simulink model "powerwindow_tl"  (R2018b)
settings: Solver=ode3  StartTime=0.0  StopTime=inf  FixedStep=0.01  RelTol=1e-3  EnableMultiTasking=on
PreLoadFcn:
  | if exist('tl_preloadfcn','file'), tl_preloadfcn(gcs,'4.4.0.41'); end
PostLoadFcn:
  | , if any(exist('dsrtsu_mdlpostloadfcn', 'file') == [2, 3, 6]), try dsrtsu_mdlpostloadfcn('Execute', bdroot); catch fprintf('Error in PostLoadFcn (dsrtsu_mdlpostloadfcn) for model "%s":\n %s\n', bdroot, lasterr); end, end,
  | if exist('tl_postloadfcn','file'), tl_postloadfcn(gcs,'4.4.0.41'); end
InitFcn:
  | if exist('tlds_init','file'), tlds_init(gcs); end
StartFcn:
  | if exist('tlds_start','file'), tlds_start(gcs); end
StopFcn:
  | if exist('tlds_stop','file'), tlds_stop(gcs); end
model workspace (MAT data in the model file):
  obs_1 = 1
  obs_10 = 1
  obs_11 = 1
  obs_12 = 1
  obs_13 = 1
  obs_14 = 1
  obs_15 = 1
  obs_16 = 1
  obs_17 = 1
  obs_18 = 1
  obs_19 = 1
  obs_2 = 1
  obs_20 = 1
  obs_21 = 1
  obs_22 = 1
  obs_23 = 1
  obs_24 = 1
  obs_25 = 1
  obs_26 = 1
  obs_27 = 1
  obs_28 = 1
  obs_29 = 1
  obs_3 = 1
  obs_30 = 1
  obs_31 = 1
  obs_32 = 1
  obs_4 = 1
  obs_5 = 1
  obs_6 = 1
  obs_7 = 1
  obs_8 = 1
  obs_9 = 1
values from neighbouring files (symbols this model uses):
  auto_down_time = 100    [start.m]
  auto_up_time = 100    [start.m]
  emergency_down_time = 100    [start.m]
  position_endstop_top = 0.4    [start.m]
undefined symbols (not defined in the file or in its folder): DiscIntNeverNeededParam
libraries: tllib x5
(part 2 of 2)

== system powerwindow_tl/PowerWindowController/Subsystem/PowerWindowController/detect_obstacle_endstop/detect_endstop ==
  window_position : Inport
  detection_ endstop_bottom : RelationalOperator  Operator=<=  OutDataTypeStr=boolean  RndMeth=Nearest  InputSameDT=on  mask(TL_RelationalOperator){data={'date',736551.40566996532}}
      settings: CopyFcn=if exist('copy_tlblock','file')==2,copy_tlblock(gcbh);end  DeleteFcn=if exist('delete_tlblock','file')==2,delete_tlblock(gcbh);end  NameChangeFcn=if exist('rename_tlblock','file')==2,rename_tlblock(gcbh);end  OpenFcn=if exist('tl_open_blockdlg','file')==2,tl_open_blockdlg(gcbh);else,open_system(gcbh,'parameter');end
      mask Help: eval(['if exist(''tl_online_help'',''file'') == 2, tl_online_help(''Topic'',''TL_RelationalOperator''),else, web([''jar:file:///'',matlabroot,''/help/toolbox/simulink/help.jar!/slref/' lower(get_param(gcbh,'Blocktype')) '.html''], ''-helpbrowser''),end'])
      mask Display:
      | [x,y] = tlDrawBrandOnBlockIcon(gcbh);
      | plot(x,y);
  detection_ endstop_top : RelationalOperator  OutDataTypeStr=boolean  RndMeth=Nearest  InputSameDT=on  mask(TL_RelationalOperator){data={'date',736551.40567012737}}
      settings: CopyFcn=if exist('copy_tlblock','file')==2,copy_tlblock(gcbh);end  DeleteFcn=if exist('delete_tlblock','file')==2,delete_tlblock(gcbh);end  NameChangeFcn=if exist('rename_tlblock','file')==2,rename_tlblock(gcbh);end  OpenFcn=if exist('tl_open_blockdlg','file')==2,tl_open_blockdlg(gcbh);else,open_system(gcbh,'parameter');end
      mask Help: eval(['if exist(''tl_online_help'',''file'') == 2, tl_online_help(''Topic'',''TL_RelationalOperator''),else, web([''jar:file:///'',matlabroot,''/help/toolbox/simulink/help.jar!/slref/' lower(get_param(gcbh,'Blocktype')) '.html''], ''-helpbrowser''),end'])
      mask Display:
      | [x,y] = tlDrawBrandOnBlockIcon(gcbh);
      | plot(x,y);
  position_ endstop_bottom : Constant  Value=0  mask(TL_Constant){data={'date',736551.40567030094}}
      settings: CopyFcn=if exist('copy_tlblock','file')==2,copy_tlblock(gcbh);end  DeleteFcn=if exist('delete_tlblock','file')==2,delete_tlblock(gcbh);end  NameChangeFcn=if exist('rename_tlblock','file')==2,rename_tlblock(gcbh);end  OpenFcn=if exist('tl_open_blockdlg','file')==2,tl_open_blockdlg(gcbh);else,open_system(gcbh,'parameter');end
      mask Help: eval(['if exist(''tl_online_help'',''file'') == 2, tl_online_help(''Topic'',''TL_Constant''),else, web([''jar:file:///'',matlabroot,''/help/toolbox/simulink/help.jar!/slref/' lower(get_param(gcbh,'Blocktype')) '.html''], ''-helpbrowser''),end'])
      mask Display:
      | [x,y] = tlDrawBrandOnBlockIcon(gcbh);
      | plot(x,y);
  position_ endstop_top : Constant  Value=position_endstop_top  mask(TL_Constant){data={'output',{'variable','position_endstop_top'},'date',736551.4102625231}}
      settings: CopyFcn=if exist('copy_tlblock','file')==2,copy_tlblock(gcbh);end  DeleteFcn=if exist('delete_tlblock','file')==2,delete_tlblock(gcbh);end  NameChangeFcn=if exist('rename_tlblock','file')==2,rename_tlblock(gcbh);end  OpenFcn=if exist('tl_open_blockdlg','file')==2,tl_open_blockdlg(gcbh);else,open_system(gcbh,'parameter');end
      mask Help: eval(['if exist(''tl_online_help'',''file'') == 2, tl_online_help(''Topic'',''TL_Constant''),else, web([''jar:file:///'',matlabroot,''/help/toolbox/simulink/help.jar!/slref/' lower(get_param(gcbh,'Blocktype')) '.html''], ''-helpbrowser''),end'])
      mask Display:
      | [x,y] = tlDrawBrandOnBlockIcon(gcbh);
      | plot(x,y);
  endstop_top : Outport
  endstop_bottom : Outport  Port=2
  wires:
  position_ endstop_top/1 -> detection_ endstop_top/2
  detection_ endstop_bottom/1 -> endstop_bottom/1  "endstop_bottom"
  detection_ endstop_top/1 -> endstop_top/1  "endstop_top"
  window_position/1 -> detection_ endstop_top/1, detection_ endstop_bottom/1
  position_ endstop_bottom/1 -> detection_ endstop_bottom/2

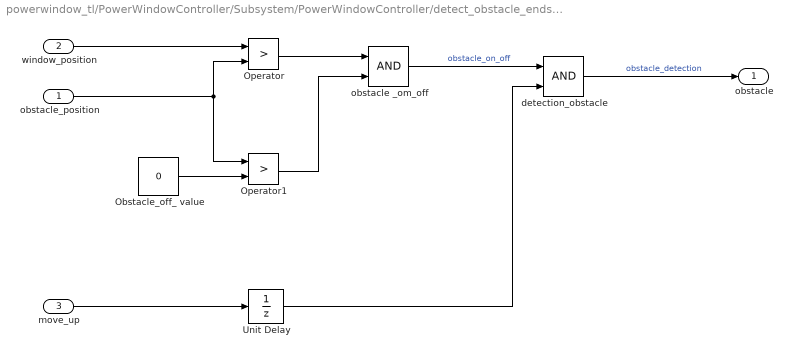
== system powerwindow_tl/PowerWindowController/Subsystem/PowerWindowController/detect_obstacle_endstop/detect_obstacle ==
  obstacle_position : Inport
  window_position : Inport  Port=2
  move_up : Inport  Port=3
  Obstacle_off_ value : Constant  Value=0  mask(TL_Constant){data={'date',736551.40567067126}}
      settings: CopyFcn=if exist('copy_tlblock','file')==2,copy_tlblock(gcbh);end  DeleteFcn=if exist('delete_tlblock','file')==2,delete_tlblock(gcbh);end  NameChangeFcn=if exist('rename_tlblock','file')==2,rename_tlblock(gcbh);end  OpenFcn=if exist('tl_open_blockdlg','file')==2,tl_open_blockdlg(gcbh);else,open_system(gcbh,'parameter');end
      mask Help: eval(['if exist(''tl_online_help'',''file'') == 2, tl_online_help(''Topic'',''TL_Constant''),else, web([''jar:file:///'',matlabroot,''/help/toolbox/simulink/help.jar!/slref/' lower(get_param(gcbh,'Blocktype')) '.html''], ''-helpbrowser''),end'])
      mask Display:
      | [x,y] = tlDrawBrandOnBlockIcon(gcbh);
      | plot(x,y);
  Operator : RelationalOperator  Operator=>  OutDataTypeStr=boolean  RndMeth=Nearest  InputSameDT=on  mask(TL_RelationalOperator){data={'date',736551.40567081014}}
      settings: CopyFcn=if exist('copy_tlblock','file')==2,copy_tlblock(gcbh);end  DeleteFcn=if exist('delete_tlblock','file')==2,delete_tlblock(gcbh);end  NameChangeFcn=if exist('rename_tlblock','file')==2,rename_tlblock(gcbh);end  OpenFcn=if exist('tl_open_blockdlg','file')==2,tl_open_blockdlg(gcbh);else,open_system(gcbh,'parameter');end
      mask Help: eval(['if exist(''tl_online_help'',''file'') == 2, tl_online_help(''Topic'',''TL_RelationalOperator''),else, web([''jar:file:///'',matlabroot,''/help/toolbox/simulink/help.jar!/slref/' lower(get_param(gcbh,'Blocktype')) '.html''], ''-helpbrowser''),end'])
      mask Display:
      | [x,y] = tlDrawBrandOnBlockIcon(gcbh);
      | plot(x,y);
  Operator1 : RelationalOperator  Operator=>  OutDataTypeStr=boolean  RndMeth=Nearest  InputSameDT=on  mask(TL_RelationalOperator){data={'date',736551.40567097219}}
      settings: CopyFcn=if exist('copy_tlblock','file')==2,copy_tlblock(gcbh);end  DeleteFcn=if exist('delete_tlblock','file')==2,delete_tlblock(gcbh);end  NameChangeFcn=if exist('rename_tlblock','file')==2,rename_tlblock(gcbh);end  OpenFcn=if exist('tl_open_blockdlg','file')==2,tl_open_blockdlg(gcbh);else,open_system(gcbh,'parameter');end
      mask Help: eval(['if exist(''tl_online_help'',''file'') == 2, tl_online_help(''Topic'',''TL_RelationalOperator''),else, web([''jar:file:///'',matlabroot,''/help/toolbox/simulink/help.jar!/slref/' lower(get_param(gcbh,'Blocktype')) '.html''], ''-helpbrowser''),end'])
      mask Display:
      | [x,y] = tlDrawBrandOnBlockIcon(gcbh);
      | plot(x,y);
  Unit Delay : UnitDelay  SampleTime=-1  mask(TL_UnitDelay){data={'output',{'variable','move_up_cmd'},'state',{'type','Bool'},'date',737383.60909223382}}
      settings: CopyFcn=if exist('copy_tlblock','file')==2,copy_tlblock(gcbh);end  DeleteFcn=if exist('delete_tlblock','file')==2,delete_tlblock(gcbh);end  NameChangeFcn=if exist('rename_tlblock','file')==2,rename_tlblock(gcbh);end  OpenFcn=if exist('tl_open_blockdlg','file')==2,tl_open_blockdlg(gcbh);else,open_system(gcbh,'parameter');end
      mask Help: eval(['if exist(''tl_online_help'',''file'') == 2, tl_online_help(''Topic'',''TL_UnitDelay''),else, web([''jar:file:///'',matlabroot,''/help/toolbox/simulink/help.jar!/slref/' lower(get_param(gcbh,'Blocktype')) '.html''], ''-helpbrowser''),end'])
      mask Display:
      | [x,y] = tlDrawBrandOnBlockIcon(gcbh);
      | plot(x,y);
  detection_obstacle : Logic  AllPortsSameDT=off  OutDataTypeStr=boolean  mask(TL_LogicalOperator){data={'date',736551.40567170142}}
      settings: CopyFcn=if exist('copy_tlblock','file')==2,copy_tlblock(gcbh);end  DeleteFcn=if exist('delete_tlblock','file')==2,delete_tlblock(gcbh);end  NameChangeFcn=if exist('rename_tlblock','file')==2,rename_tlblock(gcbh);end  OpenFcn=if exist('tl_open_blockdlg','file')==2,tl_open_blockdlg(gcbh);else,open_system(gcbh,'parameter');end
      mask Help: eval(['if exist(''tl_online_help'',''file'') == 2, tl_online_help(''Topic'',''TL_LogicalOperator''),else, web([''jar:file:///'',matlabroot,''/help/toolbox/simulink/help.jar!/slref/' lower(get_param(gcbh,'Blocktype')) '.html''], ''-helpbrowser''),end'])
      mask Display:
      | [x,y] = tlDrawBrandOnBlockIcon(gcbh);
      | plot(x,y);
  obstacle _om_off : Logic  AllPortsSameDT=off  OutDataTypeStr=boolean  mask(TL_LogicalOperator){data={'date',736551.40567187499}}
      settings: CopyFcn=if exist('copy_tlblock','file')==2,copy_tlblock(gcbh);end  DeleteFcn=if exist('delete_tlblock','file')==2,delete_tlblock(gcbh);end  NameChangeFcn=if exist('rename_tlblock','file')==2,rename_tlblock(gcbh);end  OpenFcn=if exist('tl_open_blockdlg','file')==2,tl_open_blockdlg(gcbh);else,open_system(gcbh,'parameter');end
      mask Help: eval(['if exist(''tl_online_help'',''file'') == 2, tl_online_help(''Topic'',''TL_LogicalOperator''),else, web([''jar:file:///'',matlabroot,''/help/toolbox/simulink/help.jar!/slref/' lower(get_param(gcbh,'Blocktype')) '.html''], ''-helpbrowser''),end'])
      mask Display:
      | [x,y] = tlDrawBrandOnBlockIcon(gcbh);
      | plot(x,y);
  obstacle : Outport
  wires:
  obstacle _om_off/1 -> detection_obstacle/1  "obstacle_on_off"
  Obstacle_off_ value/1 -> Operator1/2
  Operator1/1 -> obstacle _om_off/2
  detection_obstacle/1 -> obstacle/1  "obstacle_detection"
  Unit Delay/1 -> detection_obstacle/2
  obstacle_position/1 -> Operator1/1, Operator/2
  move_up/1 -> Unit Delay/1
  window_position/1 -> Operator/1
  Operator/1 -> obstacle _om_off/1

== system powerwindow_tl/PowerWindowController/Subsystem/PowerWindowController/validate_driver/check_down ==
  action : Inport
  endstop : Inport  Port=2
  allow_action : Logic  mask(TL_LogicalOperator){data={'date',736551.40567218745}}
      settings: DeleteFcn=if exist('delete_tlblock','file')==2,delete_tlblock(gcbh);end  NameChangeFcn=if exist('rename_tlblock','file')==2,rename_tlblock(gcbh);end  OpenFcn=if exist('tl_open_blockdlg','file')==2,tl_open_blockdlg(gcbh);else,open_system(gcbh,'parameter');end
      mask Help: eval(['if exist(''tl_online_help'',''file'') == 2, tl_online_help(''Topic'',''TL_LogicalOperator''),else, web([''jar:file:///'',matlabroot,''/help/toolbox/simulink/help.jar!/slref/' lower(get_param(gcbh,'Blocktype')) '.html''], ''-helpbrowser''),end'])
      mask Display: plot([-0.05, 1.05, NaN, -0.05, 1.05],[.01, .01, NaN, .99, .99])
  not : Logic  Operator=NOT  Inputs=1  mask(TL_LogicalOperator){data={'date',736551.40567231481}}
      settings: DeleteFcn=if exist('delete_tlblock','file')==2,delete_tlblock(gcbh);end  NameChangeFcn=if exist('rename_tlblock','file')==2,rename_tlblock(gcbh);end  OpenFcn=if exist('tl_open_blockdlg','file')==2,tl_open_blockdlg(gcbh);else,open_system(gcbh,'parameter');end
      mask Help: eval(['if exist(''tl_online_help'',''file'') == 2, tl_online_help(''Topic'',''TL_LogicalOperator''),else, web([''jar:file:///'',matlabroot,''/help/toolbox/simulink/help.jar!/slref/' lower(get_param(gcbh,'Blocktype')) '.html''], ''-helpbrowser''),end'])
      mask Display: plot([-0.05, 1.05, NaN, -0.05, 1.05],[.01, .01, NaN, .99, .99])
  checked_action : Outport
  wires:
  not/1 -> allow_action/2
  action/1 -> allow_action/1
  allow_action/1 -> checked_action/1  "checked_action"
  endstop/1 -> not/1

== system powerwindow_tl/PowerWindowController/Subsystem/PowerWindowController/validate_driver/check_up ==
  action : Inport
  endstop : Inport  Port=2
  allow_action : Logic  mask(TL_LogicalOperator){data={'date',736551.40567245369}}
      settings: DeleteFcn=if exist('delete_tlblock','file')==2,delete_tlblock(gcbh);end  NameChangeFcn=if exist('rename_tlblock','file')==2,rename_tlblock(gcbh);end  OpenFcn=if exist('tl_open_blockdlg','file')==2,tl_open_blockdlg(gcbh);else,open_system(gcbh,'parameter');end
      mask Help: eval(['if exist(''tl_online_help'',''file'') == 2, tl_online_help(''Topic'',''TL_LogicalOperator''),else, web([''jar:file:///'',matlabroot,''/help/toolbox/simulink/help.jar!/slref/' lower(get_param(gcbh,'Blocktype')) '.html''], ''-helpbrowser''),end'])
      mask Display: plot([-0.05, 1.05, NaN, -0.05, 1.05],[.01, .01, NaN, .99, .99])
  not : Logic  Operator=NOT  Inputs=1  mask(TL_LogicalOperator){data={'date',736551.40567262727}}
      settings: DeleteFcn=if exist('delete_tlblock','file')==2,delete_tlblock(gcbh);end  NameChangeFcn=if exist('rename_tlblock','file')==2,rename_tlblock(gcbh);end  OpenFcn=if exist('tl_open_blockdlg','file')==2,tl_open_blockdlg(gcbh);else,open_system(gcbh,'parameter');end
      mask Help: eval(['if exist(''tl_online_help'',''file'') == 2, tl_online_help(''Topic'',''TL_LogicalOperator''),else, web([''jar:file:///'',matlabroot,''/help/toolbox/simulink/help.jar!/slref/' lower(get_param(gcbh,'Blocktype')) '.html''], ''-helpbrowser''),end'])
      mask Display: plot([-0.05, 1.05, NaN, -0.05, 1.05],[.01, .01, NaN, .99, .99])
  checked_action : Outport
  wires:
  endstop/1 -> not/1
  allow_action/1 -> checked_action/1  "checked_action"
  action/1 -> allow_action/1
  not/1 -> allow_action/2

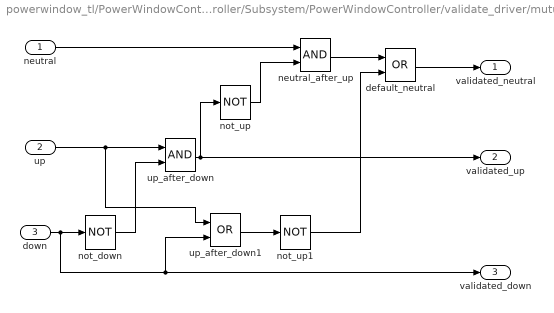
== system powerwindow_tl/PowerWindowController/Subsystem/PowerWindowController/validate_driver/mutually_exclusive ==
  neutral : Inport
  up : Inport  Port=2
  down : Inport  Port=3
  default_neutral : Logic  Operator=OR  mask(TL_LogicalOperator){data={'date',736551.40567276615}}
      settings: DeleteFcn=if exist('delete_tlblock','file')==2,delete_tlblock(gcbh);end  NameChangeFcn=if exist('rename_tlblock','file')==2,rename_tlblock(gcbh);end  OpenFcn=if exist('tl_open_blockdlg','file')==2,tl_open_blockdlg(gcbh);else,open_system(gcbh,'parameter');end
      mask Help: eval(['if exist(''tl_online_help'',''file'') == 2, tl_online_help(''Topic'',''TL_LogicalOperator''),else, web([''jar:file:///'',matlabroot,''/help/toolbox/simulink/help.jar!/slref/' lower(get_param(gcbh,'Blocktype')) '.html''], ''-helpbrowser''),end'])
      mask Display: plot([-0.05, 1.05, NaN, -0.05, 1.05],[.01, .01, NaN, .99, .99])
  neutral_after_up : Logic  mask(TL_LogicalOperator){data={'date',736551.40567293984}}
      settings: DeleteFcn=if exist('delete_tlblock','file')==2,delete_tlblock(gcbh);end  NameChangeFcn=if exist('rename_tlblock','file')==2,rename_tlblock(gcbh);end  OpenFcn=if exist('tl_open_blockdlg','file')==2,tl_open_blockdlg(gcbh);else,open_system(gcbh,'parameter');end
      mask Help: eval(['if exist(''tl_online_help'',''file'') == 2, tl_online_help(''Topic'',''TL_LogicalOperator''),else, web([''jar:file:///'',matlabroot,''/help/toolbox/simulink/help.jar!/slref/' lower(get_param(gcbh,'Blocktype')) '.html''], ''-helpbrowser''),end'])
      mask Display: plot([-0.05, 1.05, NaN, -0.05, 1.05],[.01, .01, NaN, .99, .99])
  not_down : Logic  Operator=NOT  Inputs=1  mask(TL_LogicalOperator){data={'date',736551.40567306709}}
      settings: DeleteFcn=if exist('delete_tlblock','file')==2,delete_tlblock(gcbh);end  NameChangeFcn=if exist('rename_tlblock','file')==2,rename_tlblock(gcbh);end  OpenFcn=if exist('tl_open_blockdlg','file')==2,tl_open_blockdlg(gcbh);else,open_system(gcbh,'parameter');end
      mask Help: eval(['if exist(''tl_online_help'',''file'') == 2, tl_online_help(''Topic'',''TL_LogicalOperator''),else, web([''jar:file:///'',matlabroot,''/help/toolbox/simulink/help.jar!/slref/' lower(get_param(gcbh,'Blocktype')) '.html''], ''-helpbrowser''),end'])
      mask Display: plot([-0.05, 1.05, NaN, -0.05, 1.05],[.01, .01, NaN, .99, .99])
  not_up : Logic  Operator=NOT  Inputs=1  mask(TL_LogicalOperator){data={'date',736551.40567322914}}
      settings: DeleteFcn=if exist('delete_tlblock','file')==2,delete_tlblock(gcbh);end  NameChangeFcn=if exist('rename_tlblock','file')==2,rename_tlblock(gcbh);end  OpenFcn=if exist('tl_open_blockdlg','file')==2,tl_open_blockdlg(gcbh);else,open_system(gcbh,'parameter');end
      mask Help: eval(['if exist(''tl_online_help'',''file'') == 2, tl_online_help(''Topic'',''TL_LogicalOperator''),else, web([''jar:file:///'',matlabroot,''/help/toolbox/simulink/help.jar!/slref/' lower(get_param(gcbh,'Blocktype')) '.html''], ''-helpbrowser''),end'])
      mask Display: plot([-0.05, 1.05, NaN, -0.05, 1.05],[.01, .01, NaN, .99, .99])
  not_up1 : Logic  Operator=NOT  Inputs=1  mask(TL_LogicalOperator){data={'date',736551.40567343752}}
      settings: DeleteFcn=if exist('delete_tlblock','file')==2,delete_tlblock(gcbh);end  NameChangeFcn=if exist('rename_tlblock','file')==2,rename_tlblock(gcbh);end  OpenFcn=if exist('tl_open_blockdlg','file')==2,tl_open_blockdlg(gcbh);else,open_system(gcbh,'parameter');end
      mask Help: eval(['if exist(''tl_online_help'',''file'') == 2, tl_online_help(''Topic'',''TL_LogicalOperator''),else, web([''jar:file:///'',matlabroot,''/help/toolbox/simulink/help.jar!/slref/' lower(get_param(gcbh,'Blocktype')) '.html''], ''-helpbrowser''),end'])
      mask Display: plot([-0.05, 1.05, NaN, -0.05, 1.05],[.01, .01, NaN, .99, .99])
  up_after_down : Logic  mask(TL_LogicalOperator){data={'date',736551.40567362274}}
      settings: DeleteFcn=if exist('delete_tlblock','file')==2,delete_tlblock(gcbh);end  NameChangeFcn=if exist('rename_tlblock','file')==2,rename_tlblock(gcbh);end  OpenFcn=if exist('tl_open_blockdlg','file')==2,tl_open_blockdlg(gcbh);else,open_system(gcbh,'parameter');end
      mask Help: eval(['if exist(''tl_online_help'',''file'') == 2, tl_online_help(''Topic'',''TL_LogicalOperator''),else, web([''jar:file:///'',matlabroot,''/help/toolbox/simulink/help.jar!/slref/' lower(get_param(gcbh,'Blocktype')) '.html''], ''-helpbrowser''),end'])
      mask Display: plot([-0.05, 1.05, NaN, -0.05, 1.05],[.01, .01, NaN, .99, .99])
  up_after_down1 : Logic  Operator=OR  mask(TL_LogicalOperator){data={'date',736551.40567388886}}
      settings: DeleteFcn=if exist('delete_tlblock','file')==2,delete_tlblock(gcbh);end  NameChangeFcn=if exist('rename_tlblock','file')==2,rename_tlblock(gcbh);end  OpenFcn=if exist('tl_open_blockdlg','file')==2,tl_open_blockdlg(gcbh);else,open_system(gcbh,'parameter');end
      mask Help: eval(['if exist(''tl_online_help'',''file'') == 2, tl_online_help(''Topic'',''TL_LogicalOperator''),else, web([''jar:file:///'',matlabroot,''/help/toolbox/simulink/help.jar!/slref/' lower(get_param(gcbh,'Blocktype')) '.html''], ''-helpbrowser''),end'])
      mask Display: plot([-0.05, 1.05, NaN, -0.05, 1.05],[.01, .01, NaN, .99, .99])
  validated_neutral : Outport
  validated_up : Outport  Port=2
  validated_down : Outport  Port=3
  wires:
  not_down/1 -> up_after_down/2
  up_after_down/1 -> not_up/1, validated_up/1
  not_up/1 -> neutral_after_up/2
  down/1 -> not_down/1, up_after_down1/2, validated_down/1
  neutral/1 -> neutral_after_up/1
  up/1 -> up_after_down/1, up_after_down1/1
  up_after_down1/1 -> not_up1/1
  neutral_after_up/1 -> default_neutral/1
  default_neutral/1 -> validated_neutral/1
  not_up1/1 -> default_neutral/2

== system powerwindow_tl/PowerWindowController/Subsystem/PowerWindowController/validate_passenger/check_down ==
  action : Inport
  endstop : Inport  Port=2
  allow_action : Logic  mask(TL_LogicalOperator){data={'date',736551.40567218745}}
      settings: DeleteFcn=if exist('delete_tlblock','file')==2,delete_tlblock(gcbh);end  NameChangeFcn=if exist('rename_tlblock','file')==2,rename_tlblock(gcbh);end  OpenFcn=if exist('tl_open_blockdlg','file')==2,tl_open_blockdlg(gcbh);else,open_system(gcbh,'parameter');end
      mask Help: eval(['if exist(''tl_online_help'',''file'') == 2, tl_online_help(''Topic'',''TL_LogicalOperator''),else, web([''jar:file:///'',matlabroot,''/help/toolbox/simulink/help.jar!/slref/' lower(get_param(gcbh,'Blocktype')) '.html''], ''-helpbrowser''),end'])
      mask Display: plot([-0.05, 1.05, NaN, -0.05, 1.05],[.01, .01, NaN, .99, .99])
  not : Logic  Operator=NOT  Inputs=1  mask(TL_LogicalOperator){data={'date',736551.40567231481}}
      settings: DeleteFcn=if exist('delete_tlblock','file')==2,delete_tlblock(gcbh);end  NameChangeFcn=if exist('rename_tlblock','file')==2,rename_tlblock(gcbh);end  OpenFcn=if exist('tl_open_blockdlg','file')==2,tl_open_blockdlg(gcbh);else,open_system(gcbh,'parameter');end
      mask Help: eval(['if exist(''tl_online_help'',''file'') == 2, tl_online_help(''Topic'',''TL_LogicalOperator''),else, web([''jar:file:///'',matlabroot,''/help/toolbox/simulink/help.jar!/slref/' lower(get_param(gcbh,'Blocktype')) '.html''], ''-helpbrowser''),end'])
      mask Display: plot([-0.05, 1.05, NaN, -0.05, 1.05],[.01, .01, NaN, .99, .99])
  checked_action : Outport
  wires:
  not/1 -> allow_action/2
  action/1 -> allow_action/1
  allow_action/1 -> checked_action/1  "checked_action"
  endstop/1 -> not/1

== system powerwindow_tl/PowerWindowController/Subsystem/PowerWindowController/validate_passenger/check_up ==
  action : Inport
  endstop : Inport  Port=2
  allow_action : Logic  mask(TL_LogicalOperator){data={'date',736551.40567245369}}
      settings: DeleteFcn=if exist('delete_tlblock','file')==2,delete_tlblock(gcbh);end  NameChangeFcn=if exist('rename_tlblock','file')==2,rename_tlblock(gcbh);end  OpenFcn=if exist('tl_open_blockdlg','file')==2,tl_open_blockdlg(gcbh);else,open_system(gcbh,'parameter');end
      mask Help: eval(['if exist(''tl_online_help'',''file'') == 2, tl_online_help(''Topic'',''TL_LogicalOperator''),else, web([''jar:file:///'',matlabroot,''/help/toolbox/simulink/help.jar!/slref/' lower(get_param(gcbh,'Blocktype')) '.html''], ''-helpbrowser''),end'])
      mask Display: plot([-0.05, 1.05, NaN, -0.05, 1.05],[.01, .01, NaN, .99, .99])
  not : Logic  Operator=NOT  Inputs=1  mask(TL_LogicalOperator){data={'date',736551.40567262727}}
      settings: DeleteFcn=if exist('delete_tlblock','file')==2,delete_tlblock(gcbh);end  NameChangeFcn=if exist('rename_tlblock','file')==2,rename_tlblock(gcbh);end  OpenFcn=if exist('tl_open_blockdlg','file')==2,tl_open_blockdlg(gcbh);else,open_system(gcbh,'parameter');end
      mask Help: eval(['if exist(''tl_online_help'',''file'') == 2, tl_online_help(''Topic'',''TL_LogicalOperator''),else, web([''jar:file:///'',matlabroot,''/help/toolbox/simulink/help.jar!/slref/' lower(get_param(gcbh,'Blocktype')) '.html''], ''-helpbrowser''),end'])
      mask Display: plot([-0.05, 1.05, NaN, -0.05, 1.05],[.01, .01, NaN, .99, .99])
  checked_action : Outport
  wires:
  endstop/1 -> not/1
  allow_action/1 -> checked_action/1  "checked_action"
  action/1 -> allow_action/1
  not/1 -> allow_action/2

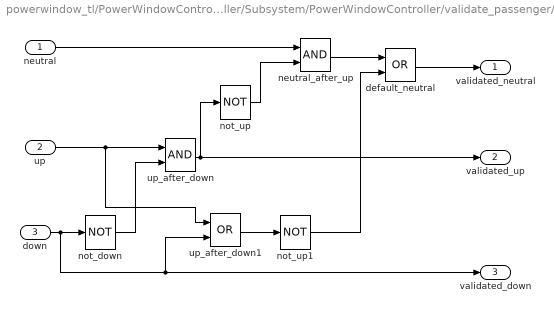
== system powerwindow_tl/PowerWindowController/Subsystem/PowerWindowController/validate_passenger/mutually_exclusive ==
  neutral : Inport
  up : Inport  Port=2
  down : Inport  Port=3
  default_neutral : Logic  Operator=OR  mask(TL_LogicalOperator){data={'date',736551.40567276615}}
      settings: DeleteFcn=if exist('delete_tlblock','file')==2,delete_tlblock(gcbh);end  NameChangeFcn=if exist('rename_tlblock','file')==2,rename_tlblock(gcbh);end  OpenFcn=if exist('tl_open_blockdlg','file')==2,tl_open_blockdlg(gcbh);else,open_system(gcbh,'parameter');end
      mask Help: eval(['if exist(''tl_online_help'',''file'') == 2, tl_online_help(''Topic'',''TL_LogicalOperator''),else, web([''jar:file:///'',matlabroot,''/help/toolbox/simulink/help.jar!/slref/' lower(get_param(gcbh,'Blocktype')) '.html''], ''-helpbrowser''),end'])
      mask Display: plot([-0.05, 1.05, NaN, -0.05, 1.05],[.01, .01, NaN, .99, .99])
  neutral_after_up : Logic  mask(TL_LogicalOperator){data={'date',736551.40567293984}}
      settings: DeleteFcn=if exist('delete_tlblock','file')==2,delete_tlblock(gcbh);end  NameChangeFcn=if exist('rename_tlblock','file')==2,rename_tlblock(gcbh);end  OpenFcn=if exist('tl_open_blockdlg','file')==2,tl_open_blockdlg(gcbh);else,open_system(gcbh,'parameter');end
      mask Help: eval(['if exist(''tl_online_help'',''file'') == 2, tl_online_help(''Topic'',''TL_LogicalOperator''),else, web([''jar:file:///'',matlabroot,''/help/toolbox/simulink/help.jar!/slref/' lower(get_param(gcbh,'Blocktype')) '.html''], ''-helpbrowser''),end'])
      mask Display: plot([-0.05, 1.05, NaN, -0.05, 1.05],[.01, .01, NaN, .99, .99])
  not_down : Logic  Operator=NOT  Inputs=1  mask(TL_LogicalOperator){data={'date',736551.40567306709}}
      settings: DeleteFcn=if exist('delete_tlblock','file')==2,delete_tlblock(gcbh);end  NameChangeFcn=if exist('rename_tlblock','file')==2,rename_tlblock(gcbh);end  OpenFcn=if exist('tl_open_blockdlg','file')==2,tl_open_blockdlg(gcbh);else,open_system(gcbh,'parameter');end
      mask Help: eval(['if exist(''tl_online_help'',''file'') == 2, tl_online_help(''Topic'',''TL_LogicalOperator''),else, web([''jar:file:///'',matlabroot,''/help/toolbox/simulink/help.jar!/slref/' lower(get_param(gcbh,'Blocktype')) '.html''], ''-helpbrowser''),end'])
      mask Display: plot([-0.05, 1.05, NaN, -0.05, 1.05],[.01, .01, NaN, .99, .99])
  not_up : Logic  Operator=NOT  Inputs=1  mask(TL_LogicalOperator){data={'date',736551.40567322914}}
      settings: DeleteFcn=if exist('delete_tlblock','file')==2,delete_tlblock(gcbh);end  NameChangeFcn=if exist('rename_tlblock','file')==2,rename_tlblock(gcbh);end  OpenFcn=if exist('tl_open_blockdlg','file')==2,tl_open_blockdlg(gcbh);else,open_system(gcbh,'parameter');end
      mask Help: eval(['if exist(''tl_online_help'',''file'') == 2, tl_online_help(''Topic'',''TL_LogicalOperator''),else, web([''jar:file:///'',matlabroot,''/help/toolbox/simulink/help.jar!/slref/' lower(get_param(gcbh,'Blocktype')) '.html''], ''-helpbrowser''),end'])
      mask Display: plot([-0.05, 1.05, NaN, -0.05, 1.05],[.01, .01, NaN, .99, .99])
  not_up1 : Logic  Operator=NOT  Inputs=1  mask(TL_LogicalOperator){data={'date',736551.40567343752}}
      settings: DeleteFcn=if exist('delete_tlblock','file')==2,delete_tlblock(gcbh);end  NameChangeFcn=if exist('rename_tlblock','file')==2,rename_tlblock(gcbh);end  OpenFcn=if exist('tl_open_blockdlg','file')==2,tl_open_blockdlg(gcbh);else,open_system(gcbh,'parameter');end
      mask Help: eval(['if exist(''tl_online_help'',''file'') == 2, tl_online_help(''Topic'',''TL_LogicalOperator''),else, web([''jar:file:///'',matlabroot,''/help/toolbox/simulink/help.jar!/slref/' lower(get_param(gcbh,'Blocktype')) '.html''], ''-helpbrowser''),end'])
      mask Display: plot([-0.05, 1.05, NaN, -0.05, 1.05],[.01, .01, NaN, .99, .99])
  up_after_down : Logic  mask(TL_LogicalOperator){data={'date',736551.40567362274}}
      settings: DeleteFcn=if exist('delete_tlblock','file')==2,delete_tlblock(gcbh);end  NameChangeFcn=if exist('rename_tlblock','file')==2,rename_tlblock(gcbh);end  OpenFcn=if exist('tl_open_blockdlg','file')==2,tl_open_blockdlg(gcbh);else,open_system(gcbh,'parameter');end
      mask Help: eval(['if exist(''tl_online_help'',''file'') == 2, tl_online_help(''Topic'',''TL_LogicalOperator''),else, web([''jar:file:///'',matlabroot,''/help/toolbox/simulink/help.jar!/slref/' lower(get_param(gcbh,'Blocktype')) '.html''], ''-helpbrowser''),end'])
      mask Display: plot([-0.05, 1.05, NaN, -0.05, 1.05],[.01, .01, NaN, .99, .99])
  up_after_down1 : Logic  Operator=OR  mask(TL_LogicalOperator){data={'date',736551.40567388886}}
      settings: DeleteFcn=if exist('delete_tlblock','file')==2,delete_tlblock(gcbh);end  NameChangeFcn=if exist('rename_tlblock','file')==2,rename_tlblock(gcbh);end  OpenFcn=if exist('tl_open_blockdlg','file')==2,tl_open_blockdlg(gcbh);else,open_system(gcbh,'parameter');end
      mask Help: eval(['if exist(''tl_online_help'',''file'') == 2, tl_online_help(''Topic'',''TL_LogicalOperator''),else, web([''jar:file:///'',matlabroot,''/help/toolbox/simulink/help.jar!/slref/' lower(get_param(gcbh,'Blocktype')) '.html''], ''-helpbrowser''),end'])
      mask Display: plot([-0.05, 1.05, NaN, -0.05, 1.05],[.01, .01, NaN, .99, .99])
  validated_neutral : Outport
  validated_up : Outport  Port=2
  validated_down : Outport  Port=3
  wires:
  not_down/1 -> up_after_down/2
  up_after_down/1 -> not_up/1, validated_up/1
  not_up/1 -> neutral_after_up/2
  down/1 -> not_down/1, up_after_down1/2, validated_down/1
  neutral/1 -> neutral_after_up/1
  up/1 -> up_after_down/1, up_after_down1/1
  up_after_down1/1 -> not_up1/1
  neutral_after_up/1 -> default_neutral/1
  default_neutral/1 -> validated_neutral/1
  not_up1/1 -> default_neutral/2

== stateflow chart powerwindow_tl/PowerWindowController/Subsystem/PowerWindowController/control ==
  settings: description=$TL$ stepfunctionclass=STATIC_FCN; date=20160819T153442; $TL$
  state systemNormal [parallel]
    settings: executionOrder=1
    state safe
      state driverNeutral
        entry:
        moveUp = 0;
        moveDown = 0;
        state passengerneutral
          entry:
          moveUp = 0;
          moveDown = 0;
          mode = 0;
        state passengerDown
          entry: moveDown = 1;
          exit: moveDown = 0;
          state iniPassengerDown
            entry:
            mode = 2;
          state autoPassengerDown
            entry:
            mode =4;
          state passengerDown
            entry:
            mode = 2;
          iniPassengerDown -> (junction 54) : after(auto_down_time,tick)
          (junction 54) -> systemNormal.safe.driverNeutral.passengerDown.passengerDown [order 2]
          (junction 54) -> autoPassengerDown [order 1] : [passenger_neutral]
        state passengerUp
          entry: moveUp = 1;
          exit: moveUp = 0;
          state iniPassengerUp
            entry:
            mode = 1;
          state PassengerUp
            entry:
            mode = 1;
          state autoPassengerUp
            entry:
            mode =3;
          iniPassengerUp -> (junction 55) : after(auto_up_time,tick)
          (junction 55) -> PassengerUp [order 2]
          (junction 55) -> autoPassengerUp [order 1] : [passenger_neutral]
        (default) -> passengerneutral
        passengerneutral -> iniPassengerUp [order 1] : [passenger_up]
        passengerneutral -> iniPassengerDown [order 2] : [passenger_down]
        PassengerUp -> passengerneutral : [passenger_neutral]
        systemNormal.safe.driverNeutral.passengerDown.passengerDown -> passengerneutral : [passenger_neutral]
        systemNormal.safe.driverNeutral.passengerDown -> passengerneutral [order 1] : [endstop_bottom]
        passengerUp -> passengerneutral [order 2] : [endstop_top]
        systemNormal.safe.driverNeutral.passengerDown -> PassengerUp [order 2] : [passenger_up]
        passengerUp -> systemNormal.safe.driverNeutral.passengerDown.passengerDown [order 1] : [passenger_down]
      state driverDown
        entry: moveDown = 1;
        exit: moveDown = 0;
        state iniDriverDown
          entry:
          mode = 2;
        state DriverDown
          entry:
          mode = 2;
        state autoDriverDown
          entry:
          mode = 4;
        iniDriverDown -> (junction 56) : after(auto_down_time,tick)
        (junction 56) -> DriverDown [order 2]
        (junction 56) -> autoDriverDown [order 1] : [driver_neutral]
      state driverUp
        entry: moveUp = 1;
        exit: moveUp = 0;
        state iniDriverUp
          entry:
          mode = 1;
        state DriverUp
          entry:
          mode =1;
        state autoDriverUp
          entry:
          mode = 3;
        iniDriverUp -> (junction 57) : after(auto_up_time,tick)
        (junction 57) -> autoDriverUp [order 1] : [driver_neutral]
        (junction 57) -> DriverUp [order 2]
      (default) -> driverNeutral
      driverNeutral -> iniDriverDown [order 3] : [driver_down]
      DriverDown -> driverNeutral : [driver_neutral]
      driverDown -> driverNeutral [order 1] : [endstop_bottom]
      DriverUp -> driverNeutral : [driver_neutral]
      driverUp -> driverNeutral [order 2] : [endstop_top]
      driverNeutral -> iniDriverUp [order 2] : [driver_up]
      driverDown -> DriverUp [order 2] : [driver_up]
      driverUp -> DriverDown [order 1] : [driver_down]
    state emergencyDown
      entry:
      moveUp = 0;
      moveDown = 1;
      mode = 5;
    state systemError
      entry:
      mode = 100;
      moveUp = 0;
      moveDown = 0;
    emergencyDown -> passengerneutral [order 2] : [endstop_bottom | after(emergency_down_time,tick)]
    (default) -> safe
    emergencyDown -> systemError [order 1] : [counter >= 100]
    driverNeutral -> emergencyDown [order 1] : [obstacle]
    safe -> systemError : [counter >= 100]
  state obstacleDetectionCounter [parallel]
    settings: executionOrder=2
    obstacleDetectionCounter -> obstacleDetectionCounter [order 2] : [obstacle]/counter = counter +1;
    obstacleDetectionCounter -> obstacleDetectionCounter [order 1] : [!obstacle]/counter = 0;
  (default) -> systemNormal [order 1]
  (default) -> obstacleDetectionCounter [order 2]
  data: auto_up_time input; auto_down_time input; emergency_down_time input; driver_neutral input boolean; driver_up input boolean; driver_down input boolean; passenger_neutral input boolean; passenger_up input boolean; passenger_down input boolean; moveDown output boolean; moveUp output boolean; obstacle input boolean; endstop_bottom input boolean; endstop_top input boolean; mode output uint8; counter local uint8
  data auto_up_time settings: description=$TL$ type=UInt8; $TL$
  data auto_down_time settings: description=$TL$ type=UInt8; $TL$
  data emergency_down_time settings: description=$TL$ type=UInt8; $TL$
  data driver_neutral settings: description=$TL$ type=Bool; $TL$
  data driver_up settings: description=$TL$ type=Bool; $TL$
  data driver_down settings: description=$TL$ type=Bool; $TL$
  data passenger_neutral settings: description=$TL$ type=Bool; $TL$
  data passenger_up settings: description=$TL$ type=Bool; $TL$
  data passenger_down settings: description=$TL$ type=Bool; $TL$
  data moveDown settings: description=$TL$ type=Bool; $TL$
  data moveUp settings: description=$TL$ type=Bool; $TL$
  data obstacle settings: description=$TL$ type=Bool; $TL$
  data endstop_bottom settings: description=$TL$ type=Bool; $TL$
  data endstop_top settings: description=$TL$ type=Bool; $TL$
  data mode settings: description=$TL$ type=UInt8; $TL$
  data counter settings: description=$TL$ type=UInt8; $TL$
